simulink model "openloop"  (R2019b)
settings: Solver=VariableStepAuto  StartTime=0.0  StopTime=35  RelTol=1e-3
values from neighbouring files (symbols this model uses):
  d_den = [L*Je L*b+R*Je+kt*ke R*b]    [SystemModel.m]
  d_num = [L*r R*r]    [SystemModel.m]
  dt = 0.2    [SystemModel.m]
  fd = fd_vec(4)    [SystemModel.m]
  p_den = [L*Je L*b+R*Je+kt*ke R*b]    [SystemModel.m]
  p_num = [kt]    [SystemModel.m]
  t_den = [1 tau]    [SystemModel.m]
  t_num = [tau]    [SystemModel.m]
  time = 15:1:30    [SystemModel.m]
  volt = 12    [SystemModel.m]
settings Model: Creator=keato  LastModifiedBy=keato

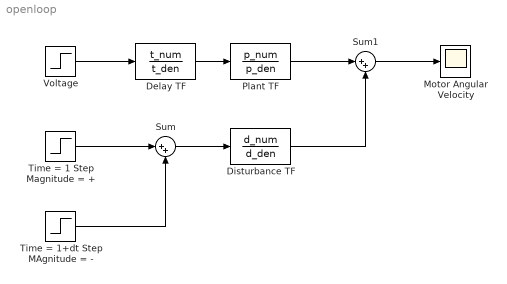
== system openloop ==
  Delay TF : TransferFcn  Numerator=t_num  Denominator=t_den
  Disturbance TF : TransferFcn  Numerator=d_num  Denominator=d_den
  Motor Angular Velocity : Scope
  Plant TF : TransferFcn  Numerator=p_num  Denominator=p_den
  Sum : Sum  Inputs=|++
  Sum1 : Sum  Inputs=|++
  Time = 1 Step Magnitude = + : Step  Time=time  After=fd  SampleTime=0
  Time = 1+dt Step MAgnitude = - : Step  Time=time+dt  After=-fd  SampleTime=0
  Voltage : Step  After=volt  SampleTime=0
  wires:
  Voltage/1 -> Delay TF/1
  Delay TF/1 -> Plant TF/1
  Plant TF/1 -> Sum1/1
  Sum1/1 -> Motor Angular Velocity/1
  Disturbance TF/1 -> Sum1/2
  Time = 1 Step Magnitude = +/1 -> Sum/1
  Sum/1 -> Disturbance TF/1
  Time = 1+dt Step MAgnitude = -/1 -> Sum/2
